simulink model "nhietdien"  (R2023b)
settings: Solver=VariableStepAuto  StartTime=0.0  StopTime=inf  RelTol=1e-3
libraries: opclib x37
settings Model: Creator=baott  LastModifiedBy=Bao

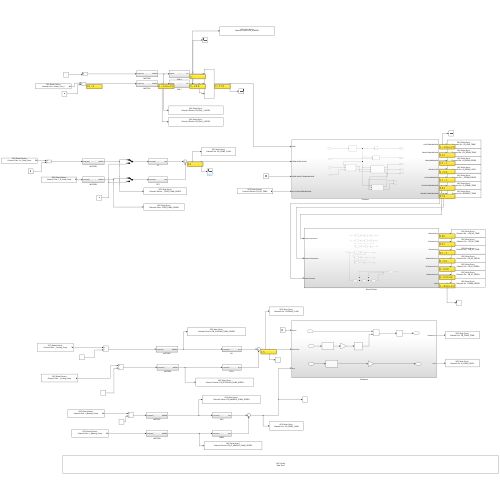
[thumbnail: Simulink's stored preview of the top-level diagram]
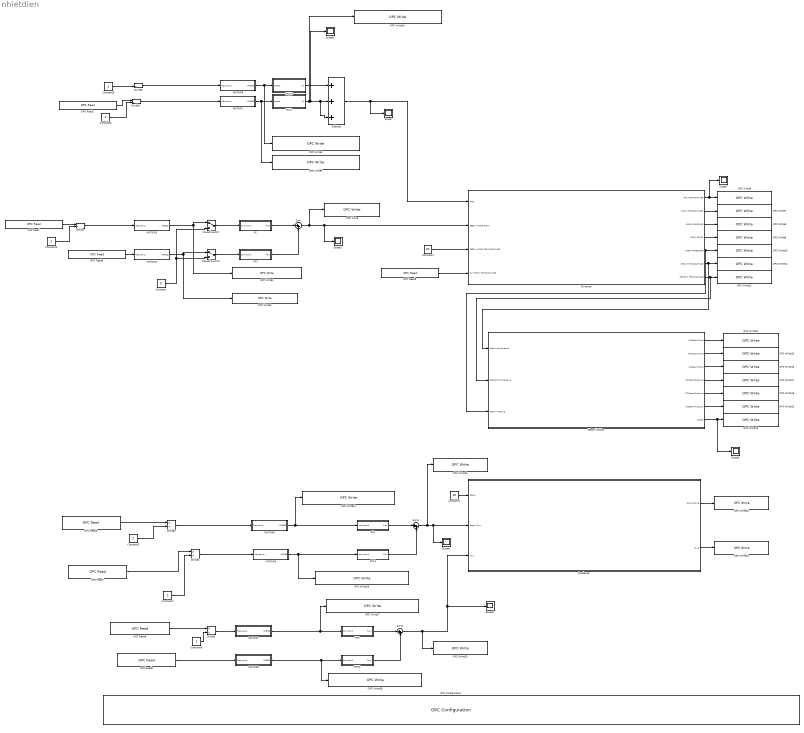
== system nhietdien ==
  CL1 : Subsystem
  Condenser : Subsystem
  Constant : Constant  Value=0
  Constant1 : Constant  Value=30
  Constant2 : Constant  Value=30
  Constant{3..6,8..9} (6 alike) : Constant  Value=2
  Divide{,1..3,5..6} (6 alike) : Product  Inputs=*/  RndMeth=Zero  SaturateOnIntegerOverflow=on
  FAN 1 : Subsystem
  FAN 3 : Subsystem
  FF : Subsystem
  Furnance : Subsystem
  MF2 : Subsystem
  MOTOR1 : Subsystem
  MOTOR3 : Subsystem
  MOTOR4 : Subsystem
  MOTOR5 : Subsystem
  MOTOR6 : Subsystem
  MOTOR7 : Subsystem
  MOTOR8 : Subsystem
  MOTOR9 : Subsystem
  Manual Switch : ManualSwitch
  Manual Switch1 : ManualSwitch
  OPC Configuration : opclib/OPC Configuration  opcServers=localhost/Kepware.KEPServerEX.V6/10  errMissingItems=Error  errReadWrite=Warn  errShutdown=Error  errRTViolation=Warn  rtEnable=on  speedup=1  showLatency=off  beingUsed=on
  OPC Read : opclib/OPC Read  serverHost=localhost  serverID=Kepware.KEPServerEX.V6  itemIDs=Channel1.Device1.Actuator_Feed_Pump  readMode=Synchronous (cache)  dataType=double  updateRate=0.5  showQual=off  showTS=off  tsMode=Seconds since start
  OPC Read1 : opclib/OPC Read  serverHost=localhost  serverID=Kepware.KEPServerEX.V6  itemIDs=Channel1.Device1.Actuator_Fan_2  readMode=Synchronous (cache)  dataType=double  updateRate=0.5  showQual=off  showTS=off  tsMode=Seconds since start
  OPC Read3 : opclib/OPC Read  serverHost=localhost  serverID=Kepware.KEPServerEX.V6  itemIDs=Channel1.Device1.FB_HP_TEMP  readMode=Synchronous (cache)  dataType=double  updateRate=0.5  showQual=off  showTS=off  tsMode=Seconds since start
  OPC Read5 : opclib/OPC Read  serverHost=localhost  serverID=Kepware.KEPServerEX.V6  itemIDs=Channel1.Device1.Actuator_Cooling_Pump  readMode=Synchronous (cache)  dataType=double  updateRate=0.5  showQual=off  showTS=off  tsMode=Seconds since start
  OPC Read6 : opclib/OPC Read  serverHost=localhost  serverID=Kepware.KEPServerEX.V6  itemIDs=Channel1.Device1.Actuator_R_Feed_Pump  readMode=Synchronous (cache)  dataType=double  updateRate=0.5  showQual=off  showTS=off  tsMode=Seconds since start
  OPC Read7 : opclib/OPC Read  serverHost=localhost  serverID=Kepware.KEPServerEX.V6  itemIDs=Channel1.Device1.Actuator_R_Cooling_Pump  readMode=Synchronous (cache)  dataType=double  updateRate=0.5  showQual=off  showTS=off  tsMode=Seconds since start
  OPC Read8 : opclib/OPC Read  serverHost=localhost  serverID=Kepware.KEPServerEX.V6  itemIDs=Channel1.Device1.Actuator_Makeup_Pump  readMode=Synchronous (cache)  dataType=double  updateRate=0.5  showQual=off  showTS=off  tsMode=Seconds since start
  OPC Read9 : opclib/OPC Read  serverHost=localhost  serverID=Kepware.KEPServerEX.V6  itemIDs=Channel1.Device1.Actuator_Makeup_Pump  readMode=Synchronous (cache)  dataType=double  updateRate=0.5  showQual=off  showTS=off  tsMode=Seconds since start
  OPC Write : opclib/OPC Write  serverHost=localhost  serverID=Kepware.KEPServerEX.V6  itemIDs=Channel1.Device1.FB_FEED_PUMP_FLOW  writeMode=Synchronous  updateRate=0
  OPC Write1 : opclib/OPC Write  serverHost=localhost  serverID=Kepware.KEPServerEX.V6  itemIDs=Channel1.Device1.FB_FEED_PUMP_SPEED  writeMode=Synchronous  updateRate=0
  OPC Write10 : opclib/OPC Write  serverHost=localhost  serverID=Kepware.KEPServerEX.V6  itemIDs=Channel1.Device1.FB_BOILER_STEAM_PRESS  writeMode=Synchronous  updateRate=0
  OPC Write11 : opclib/OPC Write  serverHost=localhost  serverID=Kepware.KEPServerEX.V6  itemIDs=Channel1.Device1.FB_BOILER_STEAM_TEMP  writeMode=Synchronous  updateRate=0
  OPC Write12 : opclib/OPC Write  serverHost=localhost  serverID=Kepware.KEPServerEX.V6  itemIDs=Channel1.Device1.FB_REHEART_TEMP  writeMode=Synchronous  updateRate=0
  OPC Write13 : opclib/OPC Write  serverHost=localhost  serverID=Kepware.KEPServerEX.V6  itemIDs=Channel1.Device1.FB_LP_PRESS  writeMode=Synchronous  updateRate=0
  OPC Write14 : opclib/OPC Write  serverHost=localhost  serverID=Kepware.KEPServerEX.V6  itemIDs=Channel1.Device1.FB_HP_TEMP  writeMode=Synchronous  updateRate=0
  OPC Write15 : opclib/OPC Write  serverHost=localhost  serverID=Kepware.KEPServerEX.V6  itemIDs=Channel1.Device1.FB_IP_TEMP  writeMode=Synchronous  updateRate=0
  OPC Write16 : opclib/OPC Write  serverHost=localhost  serverID=Kepware.KEPServerEX.V6  itemIDs=Channel1.Device1.FB_LP_TEMP  writeMode=Synchronous  updateRate=0
  OPC Write17 : opclib/OPC Write  serverHost=localhost  serverID=Kepware.KEPServerEX.V6  itemIDs=Channel1.Device1.FB_HP_PRESS  writeMode=Synchronous  updateRate=0
  OPC Write18 : opclib/OPC Write  serverHost=localhost  serverID=Kepware.KEPServerEX.V6  itemIDs=Channel1.Device1.FB_IP_PRESS  writeMode=Synchronous  updateRate=0
  OPC Write19 : opclib/OPC Write  serverHost=localhost  serverID=Kepware.KEPServerEX.V6  itemIDs=Channel1.Device1.FB_TUABIN_SPEED  writeMode=Synchronous  updateRate=0
  OPC Write2 : opclib/OPC Write  serverHost=localhost  serverID=Kepware.KEPServerEX.V6  itemIDs=Channel1.Device1.FB_R_FEED_PUMP_SPEED  writeMode=Synchronous  updateRate=0
  OPC Write20 : opclib/OPC Write  serverHost=localhost  serverID=Kepware.KEPServerEX.V6  itemIDs=Channel1.Device1.FB_COOLING_FLOW  writeMode=Synchronous  updateRate=0
  OPC Write21 : opclib/OPC Write  serverHost=localhost  serverID=Kepware.KEPServerEX.V6  itemIDs=Channel1.Device1.FB_COOLING_PUMP_SPEED  writeMode=Synchronous  updateRate=0
  OPC Write22 : opclib/OPC Write  serverHost=localhost  serverID=Kepware.KEPServerEX.V6  itemIDs=Channel1.Device1.FB_COND_TEMP  writeMode=Synchronous  updateRate=0
  OPC Write23 : opclib/OPC Write  serverHost=localhost  serverID=Kepware.KEPServerEX.V6  itemIDs=Channel1.Device1.FB_COND_LEVEL  writeMode=Synchronous  updateRate=0
  OPC Write24 : opclib/OPC Write  serverHost=localhost  serverID=Kepware.KEPServerEX.V6  itemIDs=Channel1.Device1.FB_POWER1  writeMode=Synchronous  updateRate=0
  OPC Write25 : opclib/OPC Write  serverHost=localhost  serverID=Kepware.KEPServerEX.V6  itemIDs=Channel1.Device1.FB_MAKEUP_PUMP_FLOW  writeMode=Synchronous  updateRate=0
  OPC Write26 : opclib/OPC Write  serverHost=localhost  serverID=Kepware.KEPServerEX.V6  itemIDs=Channel1.Device1.FB_RCOOLING_PUMP_SPEED  writeMode=Synchronous  updateRate=0
  OPC Write27 : opclib/OPC Write  serverHost=localhost  serverID=Kepware.KEPServerEX.V6  itemIDs=Channel1.Device1.FB_MAKEUP_PUMP_SPEED  writeMode=Synchronous  updateRate=0
  OPC Write28 : opclib/OPC Write  serverHost=localhost  serverID=Kepware.KEPServerEX.V6  itemIDs=Channel1.Device1.FB_R_MAKEUP_PUMP_SPEED  writeMode=Synchronous  updateRate=0
  OPC Write3 : opclib/OPC Write  serverHost=localhost  serverID=Kepware.KEPServerEX.V6  itemIDs=Channel1.Device1.FB_FAN_1_SPEED  writeMode=Synchronous  updateRate=0
  OPC Write5 : opclib/OPC Write  serverHost=localhost  serverID=Kepware.KEPServerEX.V6  itemIDs=Channel1.Device1.FB_FAN_2_SPEED  writeMode=Synchronous  updateRate=0
  OPC Write6 : opclib/OPC Write  serverHost=localhost  serverID=Kepware.KEPServerEX.V6  itemIDs=Channel1.Device1.FB_GAS_TEMP  writeMode=Synchronous  updateRate=0
  OPC Write7 : opclib/OPC Write  serverHost=localhost  serverID=Kepware.KEPServerEX.V6  itemIDs=Channel1.Device1.FB_DRUM_TEMP  writeMode=Synchronous  updateRate=0
  OPC Write8 : opclib/OPC Write  serverHost=localhost  serverID=Kepware.KEPServerEX.V6  itemIDs=Channel1.Device1.FB_DRUM_PRESS  writeMode=Synchronous  updateRate=0
  OPC Write9 : opclib/OPC Write  serverHost=localhost  serverID=Kepware.KEPServerEX.V6  itemIDs=Channel1.Device1.FB_DRUM_LEVEL  writeMode=Synchronous  updateRate=0
  RCL1 : Subsystem
  RF1 : Subsystem
  RMF2 : Subsystem
  Scope{,1..4,6..7} (7 alike) : Scope
  Steam Turbine : Subsystem
  Subtract : Sum  Inputs=+++
  Sum : Sum  Inputs=|++
  Sum1 : Sum  Inputs=|++
  Sum2 : Sum  Inputs=|++
  wires:
  MOTOR9/1(SPEED) -> FAN 3/1(speed), OPC Write3/1
  MOTOR1/1(SPEED) -> OPC Write5/1, FAN 1/1(speed)
  FAN 1/1(PU) -> Subtract/2, Subtract/3, Scope6/1, OPC Write24/1
  MOTOR4/1(SPEED) -> OPC Write2/1, Manual Switch1/1
  MOTOR3/1(SPEED) -> OPC Write1/1, Manual Switch/1
  Manual Switch/1 -> FF/1(command)
  Manual Switch1/1 -> RF1/1(command)
  FF/1(flow) -> Sum/1
  RF1/1(flow) -> Sum/2
  Constant/1 -> Manual Switch1/2, Manual Switch/2
  Subtract/1 -> Scope/1, Furnance/1(FIRE)
  Sum/1 -> Scope1/1, Furnance/2(FEED WATER FLOW), OPC Write/1
  OPC Read3/1 -> Furnance/4(HP STEAM TEMPURATURE)
  Constant1/1 -> Furnance/3(FEED WATER TEAMPURATURE)
  Furnance/1(GAS TEMPURATURE) -> Scope7/1, OPC Write6/1
  Furnance/2(DRUM TEMPURATURE) -> OPC Write7/1
  Furnance/3(DRUM PRESSURE) -> OPC Write8/1
  Furnance/4(DRUM LEVEL) -> OPC Write9/1
  Furnance/6(STEAM TEMPURATURE) -> Steam Turbine/1(Steam tempurature), OPC Write11/1
  Furnance/7(REHEAT TEMPURATURE) -> Steam Turbine/2(Reheart Temperature), OPC Write12/1
  Steam Turbine/7(speed) -> Scope3/1, OPC Write19/1
  Steam Turbine/1(HPSteamTemp) -> OPC Write14/1
  Steam Turbine/2(IPTSteamTemp) -> OPC Write15/1
  Steam Turbine/3(LPSteamTemp) -> OPC Write16/1
  Steam Turbine/4(HPSteamPressure) -> OPC Write17/1
  Steam Turbine/5(IPTSteamPressure) -> OPC Write18/1
  Steam Turbine/6(LPSteamPressure) -> OPC Write13/1
  CL1/1(flow) -> Sum1/1
  MOTOR6/1(SPEED) -> OPC Write26/1, RCL1/1(command)
  RCL1/1(flow) -> Sum1/2
  MOTOR5/1(SPEED) -> OPC Write21/1, CL1/1(command)
  Sum1/1 -> OPC Write20/1, Scope4/1, Condenser/2(steam flow)
  Constant2/1 -> Condenser/1(steam)
  Sum2/1 -> OPC Write25/1, Scope2/1, Condenser/3(flow)
  RMF2/1(flow) -> Sum2/2
  MF2/1(flow) -> Sum2/1
  MOTOR7/1(SPEED) -> OPC Write27/1, MF2/1(command)
  MOTOR8/1(SPEED) -> OPC Write28/1, RMF2/1(command)
  OPC Read9/1 -> MOTOR8/1(Frequency)
  Condenser/1(tempurature) -> OPC Write22/1
  Condenser/2(level) -> OPC Write23/1
  Divide/1 -> MOTOR3/1(Frequency)
  OPC Read/1 -> Divide/1
  Constant3/1 -> Divide/2
  Constant5/1 -> Divide2/2
  OPC Read5/1 -> Divide2/1
  Divide2/1 -> MOTOR5/1(Frequency)
  Constant6/1 -> Divide3/2
  OPC Read8/1 -> Divide3/1
  Divide3/1 -> MOTOR7/1(Frequency)
  Constant8/1 -> Divide5/2
  OPC Read1/1 -> Divide5/1
  OPC Read6/1 -> MOTOR4/1(Frequency)
  Divide1/1 -> MOTOR6/1(Frequency)
  OPC Read7/1 -> Divide1/1
  Constant4/1 -> Divide1/2
  Furnance/5(STEAM PRESSURE) -> Steam Turbine/3(Steam Pressure), OPC Write10/1
  Constant9/1 -> Divide6/2
  Divide6/1 -> MOTOR9/1(Frequency)
  Divide5/1 -> MOTOR1/1(Frequency)
  FAN 3/1(PU) -> Subtract/1

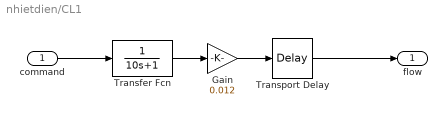
== system nhietdien/CL1 ==
  command : Inport
  Gain : Gain  Gain=0.012
  Transfer Fcn : TransferFcn  Denominator=[10, 1]
  Transport Delay : TransportDelay  DelayTime=2
  flow : Outport
  wires:
  command/1 -> Transfer Fcn/1
  Gain/1 -> Transport Delay/1
  Transport Delay/1 -> flow/1
  Transfer Fcn/1 -> Gain/1

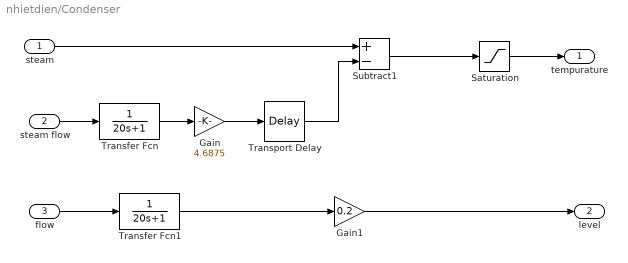
== system nhietdien/Condenser ==
  steam : Inport
  steam flow : Inport  Port=2
  flow : Inport  Port=3
  Gain : Gain  Gain=4.6875
  Gain1 : Gain  Gain=0.2
  Saturation : Saturate  UpperLimit=35  LowerLimit=25
  Subtract1 : Sum  Inputs=+-
  Transfer Fcn : TransferFcn  Denominator=[20,1]
  Transfer Fcn1 : TransferFcn  Denominator=[20,1]
  Transport Delay : TransportDelay  DelayTime=4
  tempurature : Outport
  level : Outport  Port=2
  wires:
  Transfer Fcn/1 -> Gain/1
  Subtract1/1 -> Saturation/1
  steam flow/1 -> Transfer Fcn/1
  steam/1 -> Subtract1/1
  Transport Delay/1 -> Subtract1/2
  Saturation/1 -> tempurature/1
  flow/1 -> Transfer Fcn1/1
  Gain/1 -> Transport Delay/1
  Gain1/1 -> level/1
  Transfer Fcn1/1 -> Gain1/1

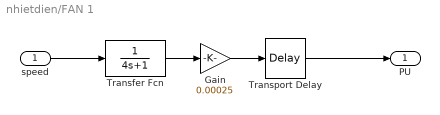
== system nhietdien/FAN 1 ==
  speed : Inport
  Gain : Gain  Gain=0.00025
  Transfer Fcn : TransferFcn  Denominator=[4, 1]
  Transport Delay : TransportDelay  DelayTime=2
  PU : Outport
  wires:
  Gain/1 -> Transport Delay/1
  Transport Delay/1 -> PU/1
  speed/1 -> Transfer Fcn/1
  Transfer Fcn/1 -> Gain/1

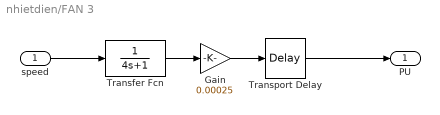
== system nhietdien/FAN 3 ==
  speed : Inport
  Gain : Gain  Gain=0.00025
  Transfer Fcn : TransferFcn  Denominator=[4, 1]
  Transport Delay : TransportDelay  DelayTime=2
  PU : Outport
  wires:
  Transfer Fcn/1 -> Gain/1
  speed/1 -> Transfer Fcn/1
  Transport Delay/1 -> PU/1
  Gain/1 -> Transport Delay/1

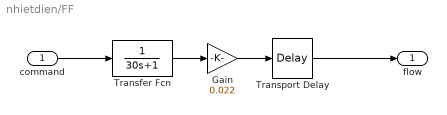
== system nhietdien/FF ==
  command : Inport
  Gain : Gain  Gain=0.022
  Transfer Fcn : TransferFcn  Denominator=[30, 1]
  Transport Delay : TransportDelay  DelayTime=3
  flow : Outport
  wires:
  command/1 -> Transfer Fcn/1
  Gain/1 -> Transport Delay/1
  Transport Delay/1 -> flow/1
  Transfer Fcn/1 -> Gain/1

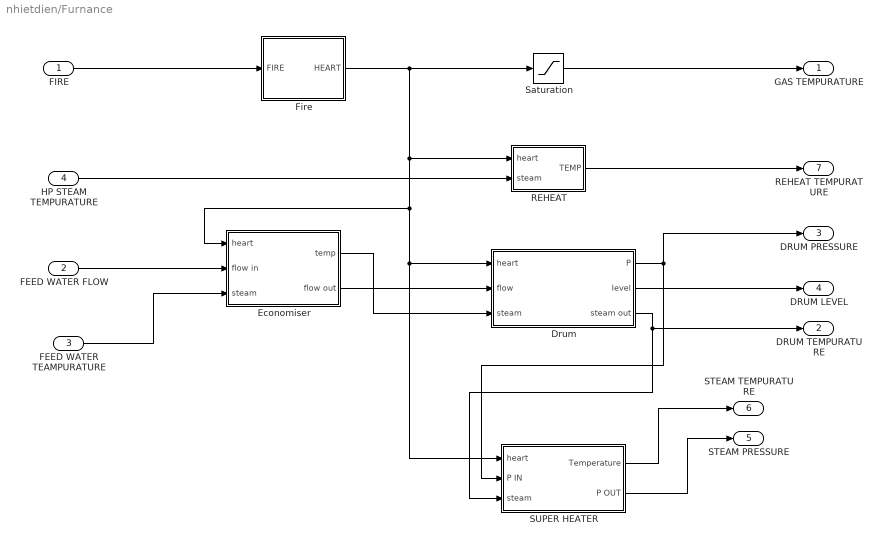
== system nhietdien/Furnance ==
  FIRE : Inport
  FEED WATER FLOW : Inport  Port=2
  FEED WATER TEAMPURATURE : Inport  Port=3
  HP STEAM TEMPURATURE : Inport  Port=4
  Drum : Subsystem
  Economiser : Subsystem
  Fire : Subsystem
  REHEAT : Subsystem
  SUPER HEATER : Subsystem
  Saturation : Saturate  UpperLimit=2000  LowerLimit=0
  GAS TEMPURATURE : Outport
  DRUM TEMPURATURE : Outport  Port=2
  DRUM PRESSURE : Outport  Port=3
  DRUM LEVEL : Outport  Port=4
  STEAM PRESSURE : Outport  Port=5
  STEAM TEMPURATURE : Outport  Port=6
  REHEAT TEMPURATURE : Outport  Port=7
  wires:
  Fire/1(HEART) -> REHEAT/1(heart), Drum/1(heart), SUPER HEATER/1(heart), Economiser/1(heart), Saturation/1
  FEED WATER FLOW/1 -> Economiser/2(flow in)
  FIRE/1 -> Fire/1(FIRE)
  HP STEAM TEMPURATURE/1 -> REHEAT/2(steam)
  Saturation/1 -> GAS TEMPURATURE/1
  Drum/2(level) -> DRUM LEVEL/1
  SUPER HEATER/1(Temperature) -> STEAM TEMPURATURE/1
  FEED WATER TEAMPURATURE/1 -> Economiser/3(steam)
  Drum/3(steam out) -> DRUM TEMPURATURE/1, SUPER HEATER/3(steam)
  SUPER HEATER/2(P OUT) -> STEAM PRESSURE/1
  Drum/1(P) -> DRUM PRESSURE/1, SUPER HEATER/2("P IN ")
  Economiser/2(flow out) -> Drum/2("flow ")
  Economiser/1(temp) -> Drum/3(steam)
  REHEAT/1(TEMP) -> REHEAT TEMPURATURE/1

== system nhietdien/MF2 ==
  command : Inport
  Gain : Gain  Gain=0.012
  Transfer Fcn : TransferFcn  Denominator=[10, 1]
  Transport Delay : TransportDelay  DelayTime=2
  flow : Outport
  wires:
  command/1 -> Transfer Fcn/1
  Gain/1 -> Transport Delay/1
  Transport Delay/1 -> flow/1
  Transfer Fcn/1 -> Gain/1

== system nhietdien/MOTOR1 ==
  Frequency : Inport
  Gain : Gain  Gain=27
  Transfer Fcn : TransferFcn  Denominator=[1, 1.1, 1]
  Transport Delay : TransportDelay  DelayTime=2
  SPEED : Outport
  wires:
  Frequency/1 -> Transfer Fcn/1
  Transfer Fcn/1 -> Gain/1
  Gain/1 -> Transport Delay/1
  Transport Delay/1 -> SPEED/1

== system nhietdien/MOTOR3 ==
  Frequency : Inport
  Gain : Gain  Gain=27
  Transfer Fcn : TransferFcn  Denominator=[1, 1.1, 1]
  Transport Delay : TransportDelay  DelayTime=2
  SPEED : Outport
  wires:
  Frequency/1 -> Transfer Fcn/1
  Transfer Fcn/1 -> Gain/1
  Gain/1 -> Transport Delay/1
  Transport Delay/1 -> SPEED/1

== system nhietdien/MOTOR4 ==
  Frequency : Inport
  Gain : Gain  Gain=27
  Transfer Fcn : TransferFcn  Denominator=[1, 1.1, 1]
  Transport Delay : TransportDelay  DelayTime=2
  SPEED : Outport
  wires:
  Transport Delay/1 -> SPEED/1
  Gain/1 -> Transport Delay/1
  Transfer Fcn/1 -> Gain/1
  Frequency/1 -> Transfer Fcn/1

== system nhietdien/MOTOR5 ==
  Frequency : Inport
  Gain : Gain  Gain=27
  Transfer Fcn : TransferFcn  Denominator=[1, 1.1, 1]
  Transport Delay : TransportDelay  DelayTime=2
  SPEED : Outport
  wires:
  Frequency/1 -> Transfer Fcn/1
  Transfer Fcn/1 -> Gain/1
  Gain/1 -> Transport Delay/1
  Transport Delay/1 -> SPEED/1

== system nhietdien/MOTOR6 ==
  Frequency : Inport
  Gain : Gain  Gain=27
  Transfer Fcn : TransferFcn  Denominator=[1, 1.1, 1]
  Transport Delay : TransportDelay  DelayTime=2
  SPEED : Outport
  wires:
  Transport Delay/1 -> SPEED/1
  Gain/1 -> Transport Delay/1
  Transfer Fcn/1 -> Gain/1
  Frequency/1 -> Transfer Fcn/1

== system nhietdien/MOTOR7 ==
  Frequency : Inport
  Gain : Gain  Gain=27
  Transfer Fcn : TransferFcn  Denominator=[1, 1.1, 1]
  Transport Delay : TransportDelay  DelayTime=2
  SPEED : Outport
  wires:
  Frequency/1 -> Transfer Fcn/1
  Transfer Fcn/1 -> Gain/1
  Gain/1 -> Transport Delay/1
  Transport Delay/1 -> SPEED/1

== system nhietdien/MOTOR8 ==
  Frequency : Inport
  Gain : Gain  Gain=27
  Transfer Fcn : TransferFcn  Denominator=[1, 1.1, 1]
  Transport Delay : TransportDelay  DelayTime=2
  SPEED : Outport
  wires:
  Transport Delay/1 -> SPEED/1
  Gain/1 -> Transport Delay/1
  Transfer Fcn/1 -> Gain/1
  Frequency/1 -> Transfer Fcn/1

== system nhietdien/MOTOR9 ==
  Frequency : Inport
  Gain : Gain  Gain=27
  Transfer Fcn : TransferFcn  Denominator=[1, 1.1, 1]
  Transport Delay : TransportDelay  DelayTime=2
  SPEED : Outport
  wires:
  Transport Delay/1 -> SPEED/1
  Gain/1 -> Transport Delay/1
  Transfer Fcn/1 -> Gain/1
  Frequency/1 -> Transfer Fcn/1

== system nhietdien/RCL1 ==
  command : Inport
  Gain : Gain  Gain=0.012
  Transfer Fcn : TransferFcn  Denominator=[10, 1]
  Transport Delay : TransportDelay  DelayTime=2
  flow : Outport
  wires:
  Transfer Fcn/1 -> Gain/1
  Transport Delay/1 -> flow/1
  Gain/1 -> Transport Delay/1
  command/1 -> Transfer Fcn/1

== system nhietdien/RF1 ==
  command : Inport
  Gain : Gain  Gain=0.022
  Transfer Fcn : TransferFcn  Denominator=[30, 1]
  Transport Delay : TransportDelay  DelayTime=3
  flow : Outport
  wires:
  Transfer Fcn/1 -> Gain/1
  Transport Delay/1 -> flow/1
  Gain/1 -> Transport Delay/1
  command/1 -> Transfer Fcn/1

== system nhietdien/RMF2 ==
  command : Inport
  Gain : Gain  Gain=0.012
  Transfer Fcn : TransferFcn  Denominator=[10, 1]
  Transport Delay : TransportDelay  DelayTime=2
  flow : Outport
  wires:
  Transfer Fcn/1 -> Gain/1
  Transport Delay/1 -> flow/1
  Gain/1 -> Transport Delay/1
  command/1 -> Transfer Fcn/1

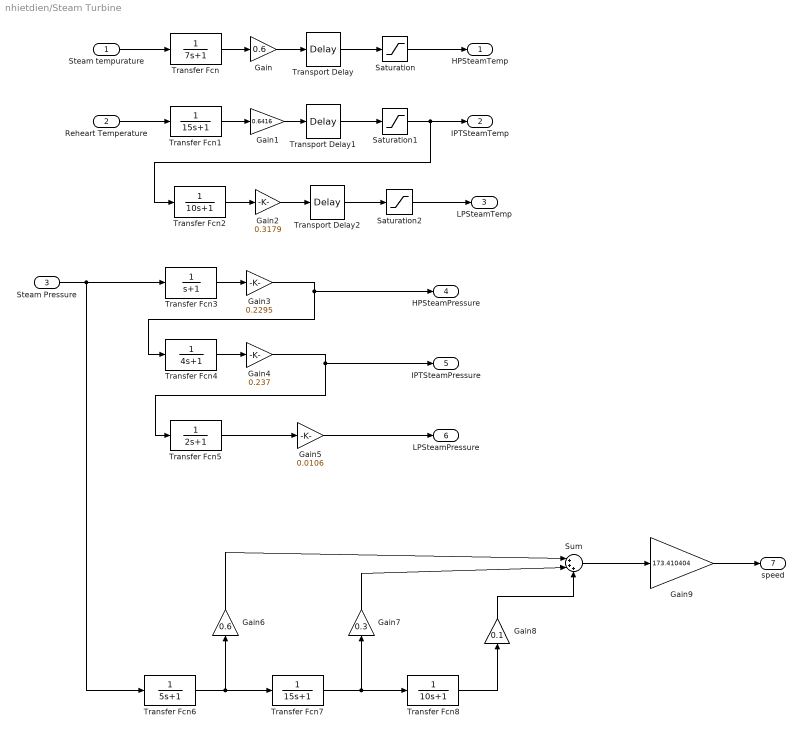
== system nhietdien/Steam Turbine ==
  Steam tempurature : Inport
  Reheart Temperature : Inport  Port=2
  Steam Pressure : Inport  Port=3
  Gain : Gain  Gain=0.6
  Gain1 : Gain  Gain=0.6416
  Gain2 : Gain  Gain=0.3179
  Gain3 : Gain  Gain=0.2295
  Gain4 : Gain  Gain=0.237
  Gain5 : Gain  Gain=0.0106
  Gain6 : Gain  Gain=0.6
  Gain7 : Gain  Gain=0.3
  Gain8 : Gain  Gain=0.1
  Gain9 : Gain  Gain=173.410404
  Saturation : Saturate  UpperLimit=100000000  LowerLimit=30
  Saturation1 : Saturate  UpperLimit=100000000  LowerLimit=30
  Saturation2 : Saturate  UpperLimit=100000000  LowerLimit=30
  Sum : Sum  Inputs=|+++
  Transfer Fcn : TransferFcn  Denominator=[7, 1]
  Transfer Fcn1 : TransferFcn  Denominator=[15, 1]
  Transfer Fcn2 : TransferFcn  Denominator=[10, 1]
  Transfer Fcn3 : TransferFcn  Denominator=[1, 1]
  Transfer Fcn4 : TransferFcn  Denominator=[4, 1]
  Transfer Fcn5 : TransferFcn  Denominator=[2, 1]
  Transfer Fcn6 : TransferFcn  Denominator=[5, 1]
  Transfer Fcn7 : TransferFcn  Denominator=[15, 1]
  Transfer Fcn8 : TransferFcn  Denominator=[10, 1]
  Transport Delay : TransportDelay  DelayTime=2
  Transport Delay1 : TransportDelay  DelayTime=2
  Transport Delay2 : TransportDelay  DelayTime=2
  HPSteamTemp : Outport
  IPTSteamTemp : Outport  Port=2
  LPSteamTemp : Outport  Port=3
  HPSteamPressure : Outport  Port=4
  IPTSteamPressure : Outport  Port=5
  LPSteamPressure : Outport  Port=6
  speed : Outport  Port=7
  wires:
  Gain2/1 -> Transport Delay2/1
  Saturation/1 -> HPSteamTemp/1
  Transfer Fcn6/1 -> Transfer Fcn7/1, Gain6/1
  Transfer Fcn3/1 -> Gain3/1
  Gain/1 -> Transport Delay/1
  Transfer Fcn1/1 -> Gain1/1
  Transfer Fcn/1 -> Gain/1
  Transport Delay/1 -> Saturation/1
  Steam tempurature/1 -> Transfer Fcn/1
  Sum/1 -> Gain9/1
  Transfer Fcn7/1 -> Gain7/1, Transfer Fcn8/1
  Transfer Fcn8/1 -> Gain8/1
  Saturation1/1 -> IPTSteamTemp/1, Transfer Fcn2/1
  Gain3/1 -> HPSteamPressure/1, Transfer Fcn4/1
  Gain8/1 -> Sum/3
  Gain5/1 -> LPSteamPressure/1
  Gain4/1 -> IPTSteamPressure/1, Transfer Fcn5/1
  Reheart Temperature/1 -> Transfer Fcn1/1
  Gain1/1 -> Transport Delay1/1
  Saturation2/1 -> LPSteamTemp/1
  Transport Delay1/1 -> Saturation1/1
  Transfer Fcn5/1 -> Gain5/1
  Transfer Fcn4/1 -> Gain4/1
  Gain7/1 -> Sum/2
  Gain6/1 -> Sum/1
  Transport Delay2/1 -> Saturation2/1
  Transfer Fcn2/1 -> Gain2/1
  Steam Pressure/1 -> Transfer Fcn6/1, Transfer Fcn3/1
  Gain9/1 -> speed/1

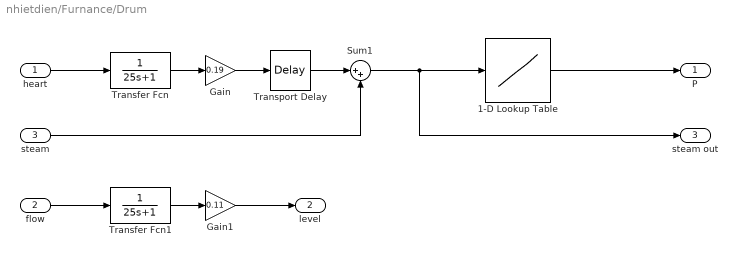
== system nhietdien/Furnance/Drum ==
  heart : Inport
  "flow " : Inport  Port=2
  steam : Inport  Port=3
  1-D Lookup Table : Lookup_n-D  NumberOfTableDimensions=1  BreakpointsForDimension1=[28.98;32.9;36.18;39.02;41.53;43.79;45.83;47.71;49.45;51.06;52.58;54;55.34;56.62;57.83;58.98;60.09;61.15;62.16;63.14;64.08;64.99;65.87;66.72;67.55;68.35;69.12;75.89;81.35;85.95;89.96;93.51;96.71;99.63;104.81;109.32;113.32;116.63;120.23;127.43;133.54;138.88;143.62;147.92;151.85;164.96;170.42;175.36;179.88;187.96;191.6;195.04;198.28;201.37;204.3;207.1;209.79;212.37;214.85;217.24;219.54;221.78;223.94;226.03;228.06;230.04;231.96;233.84;235.66;237.44;239.18;240.88;242.54;244.16;245.75;247.31;248.84;250.33;257.41;263.92;269.94;274.56;280.83;285.8;290.51;294.88;299.24;303.31;307.22;310.96;318.04;324.64;330.81;336.63;340.57;345.75;350.67;355.35;359.81;364.07;368.15;373.57;374.15]  Table=[0.004;0.005;0.006;0.007;0.008;0.009;0.01;0.011;0.012;0.013;0.014;0.015;0.016;0.017;0.018;0.019;0.02;0.021;0.022;0.023;0.024;0.025;0.026;0.027;0.028;0.029;0.03;0.04;0.05;0.06;0.07;0.08;0.09;0.1;0.12;0.14;0.16;0.18;0.2;0.25;0.3;0.35;0.4;0.5;0.6;0.7;0.8;0.9;1;1.2;1.3;1.4;1.5;1.6;1.7;1.8;1.9;2;2.1;2.2;2.3;2.4;2.5;2.6;2.7;2.8;2.9;3;3.1;3.2;3.3;3.4;3.5;3.6;3.7;3.8;3.9;4;4.5;5;5.5;6;6.5;7;7.5;8;8.5;9;9.5;10;11;12;13;14;14.7;15.7;16.7;17.7;18.6;19.6;21.6;22;22.1]  InternalRulePriority=Speed  RndMeth=Simplest
  Gain : Gain  Gain=0.19
  Gain1 : Gain  Gain=0.11
  Sum1 : Sum  Inputs=|++
  Transfer Fcn : TransferFcn  Denominator=[25, 1]
  Transfer Fcn1 : TransferFcn  Denominator=[25, 1]
  Transport Delay : TransportDelay  DelayTime=3
  P : Outport
  level : Outport  Port=2
  steam out : Outport  Port=3
  wires:
  1-D Lookup Table/1 -> P/1
  Transfer Fcn1/1 -> Gain1/1
  Gain/1 -> Transport Delay/1
  "flow "/1 -> Transfer Fcn1/1
  steam/1 -> Sum1/2
  heart/1 -> Transfer Fcn/1
  Transfer Fcn/1 -> Gain/1
  Transport Delay/1 -> Sum1/1
  Gain1/1 -> level/1
  Sum1/1 -> steam out/1, 1-D Lookup Table/1

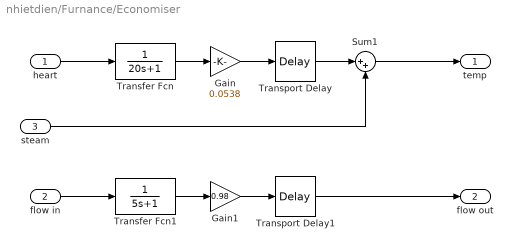
== system nhietdien/Furnance/Economiser ==
  heart : Inport
  flow in : Inport  Port=2
  steam : Inport  Port=3
  Gain : Gain  Gain=0.0538
  Gain1 : Gain  Gain=0.98
  Sum1 : Sum  Inputs=|++
  Transfer Fcn : TransferFcn  Denominator=[20, 1]
  Transfer Fcn1 : TransferFcn  Denominator=[5, 1]
  Transport Delay : TransportDelay  DelayTime=3
  Transport Delay1 : TransportDelay  DelayTime=2
  temp : Outport
  flow out : Outport  Port=2
  wires:
  Gain1/1 -> Transport Delay1/1
  steam/1 -> Sum1/2
  heart/1 -> Transfer Fcn/1
  Transport Delay1/1 -> flow out/1
  Transport Delay/1 -> Sum1/1
  Sum1/1 -> temp/1
  Gain/1 -> Transport Delay/1
  Transfer Fcn/1 -> Gain/1
  flow in/1 -> Transfer Fcn1/1
  Transfer Fcn1/1 -> Gain1/1

== system nhietdien/Furnance/Fire ==
  FIRE : Inport
  Gain : Gain  Gain=2000
  Transfer Fcn : TransferFcn  Denominator=[30,1]
  Transport Delay : TransportDelay  DelayTime=3
  HEART : Outport
  wires:
  Gain/1 -> Transport Delay/1
  FIRE/1 -> Transfer Fcn/1
  Transfer Fcn/1 -> Gain/1
  Transport Delay/1 -> HEART/1

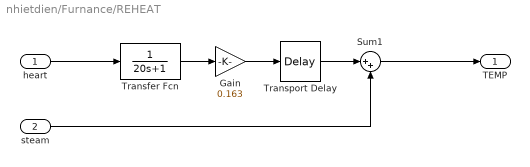
== system nhietdien/Furnance/REHEAT ==
  heart : Inport
  steam : Inport  Port=2
  Gain : Gain  Gain=0.163
  Sum1 : Sum  Inputs=|++
  Transfer Fcn : TransferFcn  Denominator=[20, 1]
  Transport Delay : TransportDelay  DelayTime=10
  TEMP : Outport
  wires:
  heart/1 -> Transfer Fcn/1
  Transfer Fcn/1 -> Gain/1
  Gain/1 -> Transport Delay/1
  Transport Delay/1 -> Sum1/1
  steam/1 -> Sum1/2
  Sum1/1 -> TEMP/1

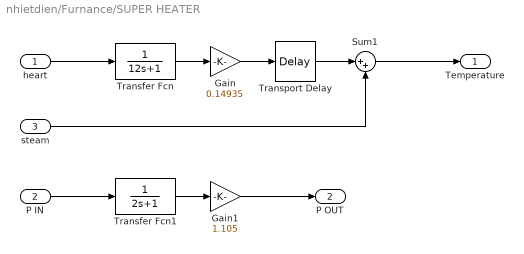
== system nhietdien/Furnance/SUPER HEATER ==
  heart : Inport
  "P IN " : Inport  Port=2
  steam : Inport  Port=3
  Gain : Gain  Gain=0.14935
  Gain1 : Gain  Gain=1.105
  Sum1 : Sum  Inputs=|++
  Transfer Fcn : TransferFcn  Denominator=[12, 1]
  Transfer Fcn1 : TransferFcn  Denominator=[2, 1]
  Transport Delay : TransportDelay
  Temperature : Outport
  P OUT : Outport  Port=2
  wires:
  Transfer Fcn/1 -> Gain/1
  steam/1 -> Sum1/2
  Gain/1 -> Transport Delay/1
  heart/1 -> Transfer Fcn/1
  Transfer Fcn1/1 -> Gain1/1
  Gain1/1 -> P OUT/1
  Transport Delay/1 -> Sum1/1
  "P IN "/1 -> Transfer Fcn1/1
  Sum1/1 -> Temperature/1
